simulink library "libMdl_multQuat"  (R2018a)
settings: Solver=VariableStepAuto  StartTime=0.0  StopTime=10.0  RelTol=1e-3
settings Model: Creator=hwinter  LastModifiedBy=Hanno

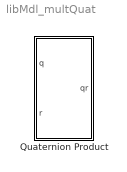
== system libMdl_multQuat ==
  Quaternion Product : Subsystem
      mask Display:
      | color('black')
      | port_label('input', 1, 'q')
      | port_label('input', 2, 'r')
      | port_label('output', 1, 'q*r')

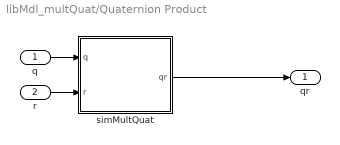
== system libMdl_multQuat/Quaternion Product ==
  q : Inport
  r : Inport  Port=2
  simMultQuat : MATLAB Function  TreatAsAtomicUnit=on
  qr : Outport
  wires:
  q/1 -> simMultQuat/1(q)
  simMultQuat/1(qr) -> qr/1
  r/1 -> simMultQuat/2(r)

== matlab function libMdl_multQuat/Quaternion Product/simMultQuat ==
  data: q input; qr output; r input
function qr = simMultQuat(q,r)

qr = multQuat(q,r);

end % function
